simulink model "4sensors in a line"  (R2019a)
settings: Solver=FixedStepAuto  StartTime=0.0  StopTime=10.0  RelTol=1e-3
undefined symbols (not defined in the file or in its folder): Battery, GYRO, LME, LRLI, MODE, MSE, PING, RME, RRLI
libraries: legoev3lib x44, simulink x19, dspstat3 x5, fuzblock x3, dspmtrx3 x3, simulink_extras x1
(part 1 of 2)
settings Model: SimulationMode=external  ExtModeTrigDuration=2  Creator=dlharr12  LastModifiedBy=juana
settings SolverCC: PositivePriorityOrder=on
settings DataIOCC: ReturnWorkspaceOutputs=off
settings OptimizationCC: PassReuseOutputArgsAs=Individual arguments  MaxStackSize=64
settings DebuggingCC: ParameterTunabilityLossMsg=error  ArithmeticOperatorsInVariantConditions=warning
settings HardwareCC: ProdBitPerPointer=32  ProdBitPerSizeT=32  ProdBitPerPtrDiffT=32  ProdLargestAtomicInteger=Long  ProdWordSize=32  ProdHWDeviceType=ARM Compatible->ARM 9  UseEmbeddedCoderFeatures=off  UseSimulinkCoderFeatures=off
settings SFSimCC: SimUseLocalCustomCode=off  MATLABDynamicMemAlloc=off
settings RTWCC: SystemTargetFile=ert.tlc  HardwareBoard=LEGO MINDSTORMS EV3  TLCOptions="-aInlineSetEventsForThisBaseRateFcn=TLC_FALSE -aSuppressMultiTaskScheduler=TLC_FALSE  -aRateBasedStepFcn=0"  TemplateMakefile=ert_default_tmf  GenerateReport=on  RTWUseLocalCustomCode=off  Toolchain=Sourcery G++ Lite v2009q3  IncludeHyperlinkInReport=on  LaunchReport=on  GenerateTraceInfo=on  GenerateTraceReport=on  GenerateTraceReportSl=on  GenerateTraceReportSf=on  GenerateTraceReportEml=on
settings CodeAppCC: ForceParamTrailComments=on  IgnoreCustomStorageClasses=off  OperatorAnnotations=on  SimulinkDataObjDesc=on  SFDataObjDesc=on  InsertBlockDesc=on
settings ERTTargetCC: SupportContinuousTime=on  SupportNonInlinedSFcns=on  SupportVariableSizeSignals=on

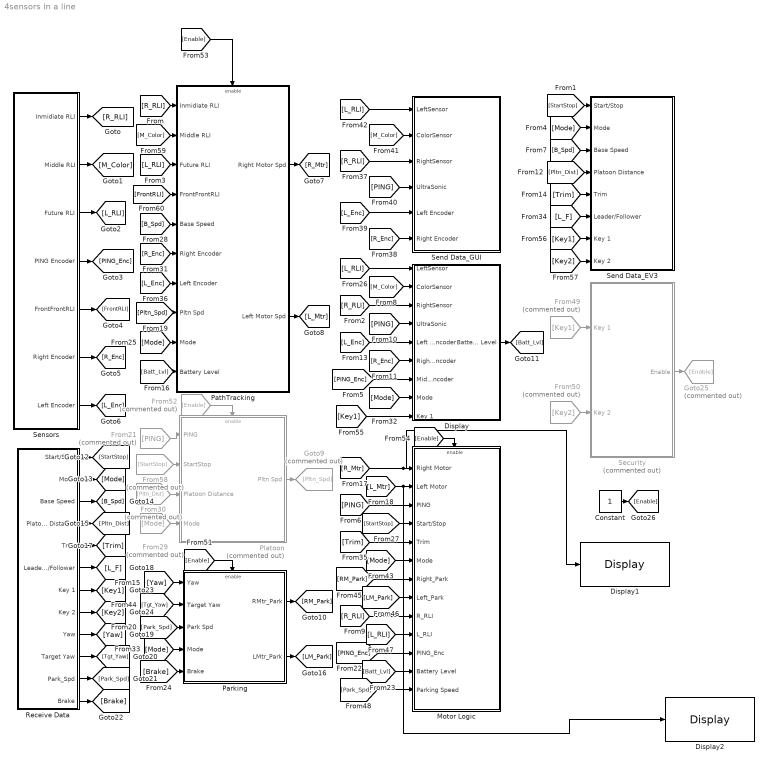
== system 4sensors in a line ==
  Constant : Constant
  Display : Subsystem
  Display1 : legoev3lib/Display  slcdStr=Rightm2  slcdLine=5  slcdFormat=Decimal
      settings: SourceProductName=Simulink Support Package for LEGO MINDSTORMS EV3 Hardware  SourceProductBaseCode=LEGOEV3
  Display2 : legoev3lib/Display  slcdStr=Leftm2  slcdLine=6  slcdFormat=Decimal
      settings: SourceProductName=Simulink Support Package for LEGO MINDSTORMS EV3 Hardware  SourceProductBaseCode=LEGOEV3
  From21 : From  Commented=on  GotoTag=PING
  From29 : From  Commented=on  GotoTag=Mode
  From30 : From  Commented=on  GotoTag=Pltn_Dist
  From49 : From  Commented=on  GotoTag=Key1
  From50 : From  Commented=on  GotoTag=Key2
  From52 : From  Commented=on  GotoTag=Enable
  From58 : From  Commented=on  GotoTag=StartStop
  Goto25 : Goto  Commented=on  GotoTag=Enable
  Goto9 : Goto  Commented=on  GotoTag=Pltn_Spd
  Motor Logic : Subsystem
  Parking : Subsystem
  PathTracking : Subsystem
  Platoon : Subsystem  Commented=on
  Receive Data : Subsystem
  Security : Subsystem  Commented=on
  Send Data_EV3 : Subsystem
  Send Data_GUI : Subsystem
  Sensors : Subsystem
  wires:
  Sensors/1(Inmidiate RLI) -> [R_RLI]
  Sensors/2(Middle RLI) -> [M_Color]
  Sensors/3(Future RLI) -> [L_RLI]
  Sensors/4(PING Encoder) -> [PING_Enc]
  Sensors/5(FrontFrontRLI) -> [FrontRLI]
  Sensors/6(Right Encoder) -> [R_Enc]
  Sensors/7(Left Encoder) -> [L_Enc]
  [R_Mtr] -> Display1/1, Motor Logic/1(Right Motor)
  [PING] -> Motor Logic/3(PING)
  [StartStop] -> Motor Logic/4(Start/Stop)
  Receive Data/2(Mode) -> [Mode]
  Receive Data/3(Base Speed) -> [B_Spd]
  Receive Data/4(Platoon Distance) -> [Pltn_Dist]
  [B_Spd] -> PathTracking/5(Base Speed)
  PathTracking/2(Left Motor Spd) -> [L_Mtr]
  From30/1 -> Platoon/3(Platoon Distance)
  Platoon/1(Pltn Spd) -> Goto9/1
  From29/1 -> Platoon/4(Mode)
  [L_RLI] -> PathTracking/3(Future RLI)
  [PING_Enc] -> Motor Logic/11(PING_Enc)
  From21/1 -> Platoon/1(PING)
  PathTracking/1(Right Motor Spd) -> [R_Mtr]
  [R_RLI] -> PathTracking/1(Inmidiate RLI)
  [R_Enc] -> Display/6(Right Encoder)
  [L_Enc] -> Display/5(Left Encoder)
  [PING] -> Display/4(UltraSonic)
  [L_RLI] -> Display/1(LeftSensor)
  [M_Color] -> Display/2(ColorSensor)
  [PING_Enc] -> Display/7(Middle Encoder)
  [R_RLI] -> Display/3(RightSensor)
  [Mode] -> Display/8(Mode)
  Receive Data/5(Trim) -> [Trim]
  [Trim] -> Motor Logic/5(Trim)
  [R_Enc] -> PathTracking/6(Right Encoder)
  [L_Enc] -> PathTracking/7(Left Encoder)
  [Pltn_Spd] -> PathTracking/8(Pltn Spd)
  [Mode] -> PathTracking/9(Mode)
  [R_Enc] -> Send Data_GUI/6(Right Encoder)
  [PING] -> Send Data_GUI/4(UltraSonic)
  [L_Enc] -> Send Data_GUI/5(Left Encoder)
  [R_RLI] -> Send Data_GUI/3(RightSensor)
  [M_Color] -> Send Data_GUI/2(ColorSensor)
  [L_RLI] -> Send Data_GUI/1(LeftSensor)
  [Mode] -> Motor Logic/6(Mode)
  Receive Data/6(Leader/Follower) -> [L_F]
  Parking/1(RMtr_Park) -> [RM_Park]
  Parking/2(LMtr_Park) -> [LM_Park]
  [RM_Park] -> Motor Logic/7(Right_Park)
  [LM_Park] -> Motor Logic/8(Left_Park)
  Receive Data/9(Yaw) -> [Yaw]
  Receive Data/10(Target Yaw) -> [Tgt_Yaw]
  [Yaw] -> Parking/1(Yaw)
  [Tgt_Yaw] -> Parking/2(Target Yaw)
  [Mode] -> Parking/4(Mode)
  [StartStop] -> Send Data_EV3/1(Start/Stop)
  [Mode] -> Send Data_EV3/2(Mode)
  [B_Spd] -> Send Data_EV3/3(Base Speed)
  [Pltn_Dist] -> Send Data_EV3/4(Platoon Distance)
  [Trim] -> Send Data_EV3/5(Trim)
  [L_F] -> Send Data_EV3/6(Leader/Follower)
  [R_RLI] -> Motor Logic/9(R_RLI)
  [L_RLI] -> Motor Logic/10(L_RLI)
  Display/1(Battery Level) -> [Batt_Lvl]
  [Batt_Lvl] -> PathTracking/10(Battery Level)
  Receive Data/11(Park_Spd) -> [Park_Spd]
  [Park_Spd] -> Parking/3(Park Spd)
  [Batt_Lvl] -> Motor Logic/12(Battery Level)
  Receive Data/12(Brake) -> [Brake]
  [Brake] -> Parking/5(Brake)
  [Park_Spd] -> Motor Logic/13(Parking Speed)
  Receive Data/7(Key 1) -> [Key1]
  Receive Data/8(Key 2) -> [Key2]
  From50/1 -> Security/2(Key 2)
  From49/1 -> Security/1(Key 1)
  Security/1(Enable) -> Goto25/1
  [Enable] -> Parking/Enable
  From52/1 -> Platoon/Enable
  [Enable] -> PathTracking/Enable
  [Enable] -> Motor Logic/Enable
  Receive Data/1(Start/Stop) -> [StartStop]
  [Key1] -> Display/9(Key 1)
  [Key1] -> Send Data_EV3/7(Key 1)
  [Key2] -> Send Data_EV3/8(Key 2)
  From58/1 -> Platoon/2(StartStop)
  Constant/1 -> [Enable]
  [M_Color] -> PathTracking/2(Middle RLI)
  [FrontRLI] -> PathTracking/4(FrontFrontRLI)
  [L_Mtr] -> Display2/1, Motor Logic/2(Left Motor)

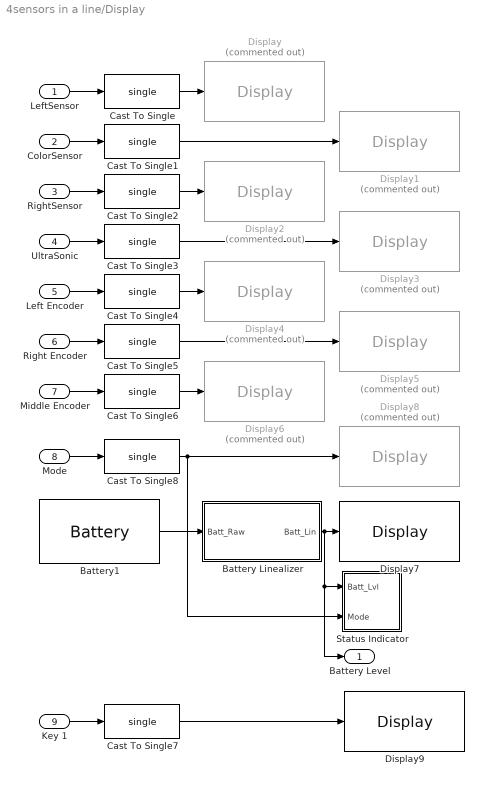
== system 4sensors in a line/Display ==
  LeftSensor : Inport
  ColorSensor : Inport  Port=2
  RightSensor : Inport  Port=3
  UltraSonic : Inport  Port=4
  Left Encoder : Inport  Port=5
  Right Encoder : Inport  Port=6
  Middle Encoder : Inport  Port=7
  Mode : Inport  Port=8
  Key 1 : Inport  Port=9
  Battery Linealizer : Subsystem
  Battery1 : legoev3lib/Battery  SampleTime=0.5
      settings: SourceProductName=Simulink Support Package for LEGO MINDSTORMS EV3 Hardware  SourceProductBaseCode=LEGOEV3
  Cast To Single{,1..8} (9 alike) : DataTypeConversion  OutDataTypeStr=single
  Display : legoev3lib/Display  Commented=on  slcdStr=LRLI:  slcdLine=1  slcdFormat=Decimal
      settings: SourceProductName=Simulink Support Package for LEGO MINDSTORMS EV3 Hardware  SourceProductBaseCode=LEGOEV3
  Display1 : legoev3lib/Display  Commented=on  slcdStr=GYRO:  slcdLine=2  slcdFormat=Decimal
      settings: SourceProductName=Simulink Support Package for LEGO MINDSTORMS EV3 Hardware  SourceProductBaseCode=LEGOEV3
  Display2 : legoev3lib/Display  Commented=on  slcdStr=RRLI:  slcdLine=3  slcdFormat=Decimal
      settings: SourceProductName=Simulink Support Package for LEGO MINDSTORMS EV3 Hardware  SourceProductBaseCode=LEGOEV3
  Display3 : legoev3lib/Display  Commented=on  slcdStr=PING:  slcdLine=4  slcdFormat=Decimal
      settings: SourceProductName=Simulink Support Package for LEGO MINDSTORMS EV3 Hardware  SourceProductBaseCode=LEGOEV3
  Display4 : legoev3lib/Display  Commented=on  slcdStr=LME:  slcdLine=5  slcdFormat=Decimal
      settings: SourceProductName=Simulink Support Package for LEGO MINDSTORMS EV3 Hardware  SourceProductBaseCode=LEGOEV3
  Display5 : legoev3lib/Display  Commented=on  slcdStr=RME:  slcdLine=6  slcdFormat=Decimal
      settings: SourceProductName=Simulink Support Package for LEGO MINDSTORMS EV3 Hardware  SourceProductBaseCode=LEGOEV3
  Display6 : legoev3lib/Display  Commented=on  slcdStr=MSE:  slcdLine=7  slcdFormat=Decimal
      settings: SourceProductName=Simulink Support Package for LEGO MINDSTORMS EV3 Hardware  SourceProductBaseCode=LEGOEV3
  Display7 : legoev3lib/Display  slcdStr=Battery:  slcdLine=9  slcdFormat=Decimal
      settings: SourceProductName=Simulink Support Package for LEGO MINDSTORMS EV3 Hardware  SourceProductBaseCode=LEGOEV3
  Display8 : legoev3lib/Display  Commented=on  slcdStr=MODE:  slcdLine=8  slcdFormat=Decimal
      settings: SourceProductName=Simulink Support Package for LEGO MINDSTORMS EV3 Hardware  SourceProductBaseCode=LEGOEV3
  Display9 : legoev3lib/Display  slcdStr=Key 1:  slcdLine=10  slcdFormat=Decimal
      settings: SourceProductName=Simulink Support Package for LEGO MINDSTORMS EV3 Hardware  SourceProductBaseCode=LEGOEV3
  Status Indicator : Subsystem
  Battery Level : Outport
  wires:
  ColorSensor/1 -> Cast To Single1/1
  LeftSensor/1 -> Cast To Single/1
  RightSensor/1 -> Cast To Single2/1
  UltraSonic/1 -> Cast To Single3/1
  Left Encoder/1 -> Cast To Single4/1
  Right Encoder/1 -> Cast To Single5/1
  Middle Encoder/1 -> Cast To Single6/1
  Cast To Single/1 -> Display/1
  Cast To Single1/1 -> Display1/1
  Cast To Single2/1 -> Display2/1
  Cast To Single3/1 -> Display3/1
  Cast To Single4/1 -> Display4/1
  Cast To Single5/1 -> Display5/1
  Cast To Single6/1 -> Display6/1
  Mode/1 -> Cast To Single8/1
  Cast To Single8/1 -> Status Indicator/2(Mode), Display8/1
  Battery1/1 -> Battery Linealizer/1(Batt_Raw)
  Battery Linealizer/1(Batt_Lin) -> Display7/1, Battery Level/1, Status Indicator/1(Batt_Lvl)
  Key 1/1 -> Cast To Single7/1
  Cast To Single7/1 -> Display9/1

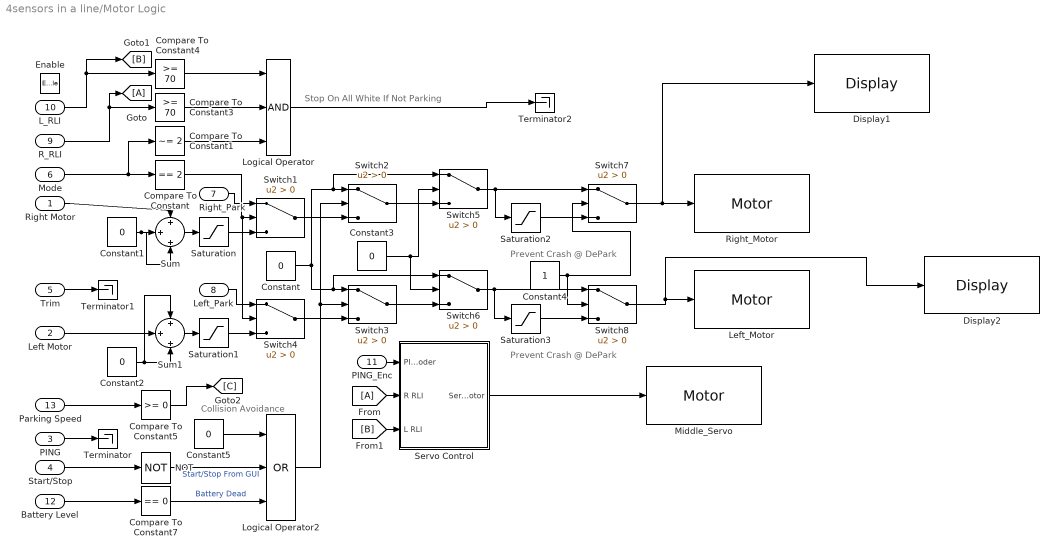
== system 4sensors in a line/Motor Logic ==
  note: Prevent Crash @ DePark
  note: Collision Avoidance
  note: Stop On All White If Not Parking
  note: Prevent Crash @ DePark
  Right Motor : Inport
  Left Motor : Inport  Port=2
  PING : Inport  Port=3
  Start/Stop : Inport  Port=4
  Trim : Inport  Port=5
  Mode : Inport  Port=6
  Right_Park : Inport  Port=7
  Left_Park : Inport  Port=8
  R_RLI : Inport  Port=9
  L_RLI : Inport  Port=10
  PING_Enc : Inport  Port=11
  Battery Level : Inport  Port=12
  Parking Speed : Inport  Port=13
  Enable : EnablePort
  Compare To Constant : simulink/Logic and Bit Operations/Compare To Constant  relop===  const=2  OutDataTypeStr=boolean
  Compare To Constant1 : simulink/Logic and Bit Operations/Compare To Constant  relop=~=  const=2  OutDataTypeStr=boolean
  Compare To Constant3 : simulink/Logic and Bit Operations/Compare To Constant  relop=>=  const=70  OutDataTypeStr=boolean
  Compare To Constant4 : simulink/Logic and Bit Operations/Compare To Constant  relop=>=  const=70  OutDataTypeStr=boolean
  Compare To Constant5 : simulink/Logic and Bit Operations/Compare To Constant  relop=>=  const=0  OutDataTypeStr=boolean
  Compare To Constant7 : simulink/Logic and Bit Operations/Compare To Constant  relop===  const=0  OutDataTypeStr=boolean
  Constant{,1..3,5} (5 alike) : Constant  Value=0
  Constant4 : Constant
  Display1 : legoev3lib/Display  slcdStr=Rightm3  slcdLine=7  slcdFormat=Decimal
      settings: SourceProductName=Simulink Support Package for LEGO MINDSTORMS EV3 Hardware  SourceProductBaseCode=LEGOEV3
  Display2 : legoev3lib/Display  slcdStr=Leftm3  slcdLine=8  slcdFormat=Decimal
      settings: SourceProductName=Simulink Support Package for LEGO MINDSTORMS EV3 Hardware  SourceProductBaseCode=LEGOEV3
  Left_Motor : legoev3lib/Motor  sportNumber=D  sstopAction=Brake
  Logical Operator : Logic  Inputs=3  AllPortsSameDT=off  OutDataTypeStr=boolean
  Logical Operator2 : Logic  Operator=OR  Inputs=3  AllPortsSameDT=off  OutDataTypeStr=boolean
  Middle_Servo : legoev3lib/Motor  sportNumber=C  sstopAction=Brake
  NOT : Logic  Operator=NOT  IconShape=distinctive  AllPortsSameDT=off  OutDataTypeStr=boolean
  Right_Motor : legoev3lib/Motor  sportNumber=A  sstopAction=Brake
  Saturation : Saturate  UpperLimit=100  LowerLimit=-100
  Saturation1 : Saturate  UpperLimit=100  LowerLimit=-100
  Saturation2 : Saturate  UpperLimit=0  LowerLimit=-100
  Saturation3 : Saturate  UpperLimit=0  LowerLimit=-100
  Servo Control : Subsystem
  Sum : Sum  Inputs=+|+|+
  Sum1 : Sum  Inputs=+|+|+
  Switch{1..8} (8 alike) : Switch  Criteria=u2 > Threshold
  Terminator : Terminator
  Terminator1 : Terminator
  Terminator2 : Terminator
  wires:
  Sum1/1 -> Saturation1/1
  Start/Stop/1 -> NOT/1
  NOT/1 -> Logical Operator2/2  "Start/Stop From GUI"
  Right Motor/1 -> Sum/1
  Sum/1 -> Saturation/1
  Left Motor/1 -> Sum1/2
  Mode/1 -> Compare To Constant1/1, Compare To Constant/1
  Saturation/1 -> Switch1/3
  Saturation1/1 -> Switch4/3
  Compare To Constant/1 -> Switch4/2, Switch1/2
  Right_Park/1 -> Switch1/1
  Left_Park/1 -> Switch4/1
  Logical Operator2/1 -> Switch3/2, Switch2/2
  Switch1/1 -> Switch2/3
  Switch4/1 -> Switch3/3
  Constant/1 -> Switch5/1, Switch2/1, Switch6/1, Switch3/1
  Constant1/1 -> Sum/3, Sum/2
  Constant2/1 -> Sum1/1, Sum1/3
  Switch2/1 -> Switch5/3
  Switch3/1 -> Switch6/3
  L_RLI/1 -> [B], Compare To Constant4/1
  R_RLI/1 -> [A], Compare To Constant3/1
  Servo Control/1(Servo Motor) -> Middle_Servo/1
  PING_Enc/1 -> Servo Control/1(PING Encoder)
  [A] -> Servo Control/2(R RLI)
  [B] -> Servo Control/3(L RLI)
  Compare To Constant1/1 -> Logical Operator/3
  Compare To Constant3/1 -> Logical Operator/2
  Compare To Constant4/1 -> Logical Operator/1
  Logical Operator/1 -> Terminator2/1
  Battery Level/1 -> Compare To Constant7/1
  Compare To Constant7/1 -> Logical Operator2/3  "Battery Dead"
  PING/1 -> Terminator/1
  Compare To Constant5/1 -> [C]
  Parking Speed/1 -> Compare To Constant5/1
  Saturation2/1 -> Switch7/3
  Switch8/1 -> Display2/1, Left_Motor/1
  Switch5/1 -> Saturation2/1, Switch7/1
  Saturation3/1 -> Switch8/3
  Constant4/1 -> Switch8/2, Switch7/2
  Switch6/1 -> Saturation3/1, Switch8/1
  Trim/1 -> Terminator1/1
  Constant3/1 -> Switch6/2, Switch5/2
  Constant5/1 -> Logical Operator2/1
  Switch7/1 -> Display1/1, Right_Motor/1

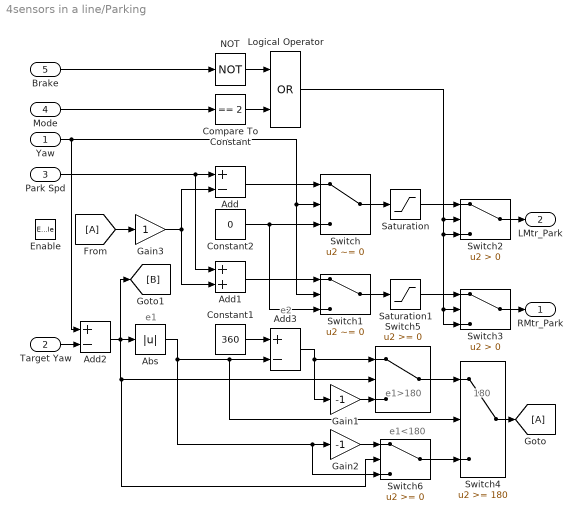
== system 4sensors in a line/Parking ==
  note: e1
  note: e2
  note: e1<180
  note: e1>180
  note: 180
  Yaw : Inport
  Target Yaw : Inport  Port=2
  Park Spd : Inport  Port=3
  Mode : Inport  Port=4
  Brake : Inport  Port=5
  Enable : EnablePort
  Abs : Abs
  Add : Sum  Inputs=+-
  Add1 : Sum
  Add2 : Sum  Inputs=+-
  Add3 : Sum  Inputs=+-
  Compare To Constant : simulink/Logic and Bit Operations/Compare To Constant  relop===  const=2  OutDataTypeStr=boolean
  Constant1 : Constant  Value=360
  Constant2 : Constant  Value=0
  Gain1 : Gain  Gain=-1
  Gain2 : Gain  Gain=-1
  Gain3 : Gain
  Logical Operator : Logic  Operator=OR  AllPortsSameDT=off  OutDataTypeStr=boolean
  NOT : Logic  Operator=NOT  IconShape=distinctive  AllPortsSameDT=off  OutDataTypeStr=boolean
  Saturation : Saturate  UpperLimit=60  LowerLimit=-60
  Saturation1 : Saturate  UpperLimit=60  LowerLimit=-60
  Switch : Switch  Criteria=u2 ~= 0
  Switch1 : Switch  Criteria=u2 ~= 0
  Switch2 : Switch  Criteria=u2 > Threshold
  Switch3 : Switch  Criteria=u2 > Threshold
  Switch4 : Switch  Threshold=180
  Switch5 : Switch
  Switch6 : Switch
  RMtr_Park : Outport
  LMtr_Park : Outport  Port=2
  wires:
  Mode/1 -> Compare To Constant/1
  Gain2/1 -> Switch6/1
  Target Yaw/1 -> Add2/2
  Add3/1 -> Gain1/1, Switch5/1
  Switch5/1 -> Switch4/1
  Switch6/1 -> Switch4/3
  Park Spd/1 -> Add1/1, Add/1
  Gain1/1 -> Switch5/3
  Gain3/1 -> Add/2, Add1/2
  Add2/1 -> [B], Switch6/2, Switch5/2, Abs/1
  Add/1 -> Switch/1
  Constant1/1 -> Add3/1
  Abs/1 -> Gain2/1, Switch6/3, Switch4/2, Add3/2
  Add1/1 -> Switch1/1
  Constant2/1 -> Switch1/3, Switch/3
  Yaw/1 -> Add2/1, Switch1/2, Switch/2
  Switch4/1 -> [A]
  [A] -> Gain3/1
  Switch2/1 -> LMtr_Park/1
  Switch3/1 -> RMtr_Park/1
  Compare To Constant/1 -> Logical Operator/2
  Logical Operator/1 -> Switch2/2, Switch2/3, Switch3/3, Switch3/2
  Brake/1 -> NOT/1
  NOT/1 -> Logical Operator/1
  Saturation/1 -> Switch2/1
  Saturation1/1 -> Switch3/1
  Switch/1 -> Saturation/1
  Switch1/1 -> Saturation1/1

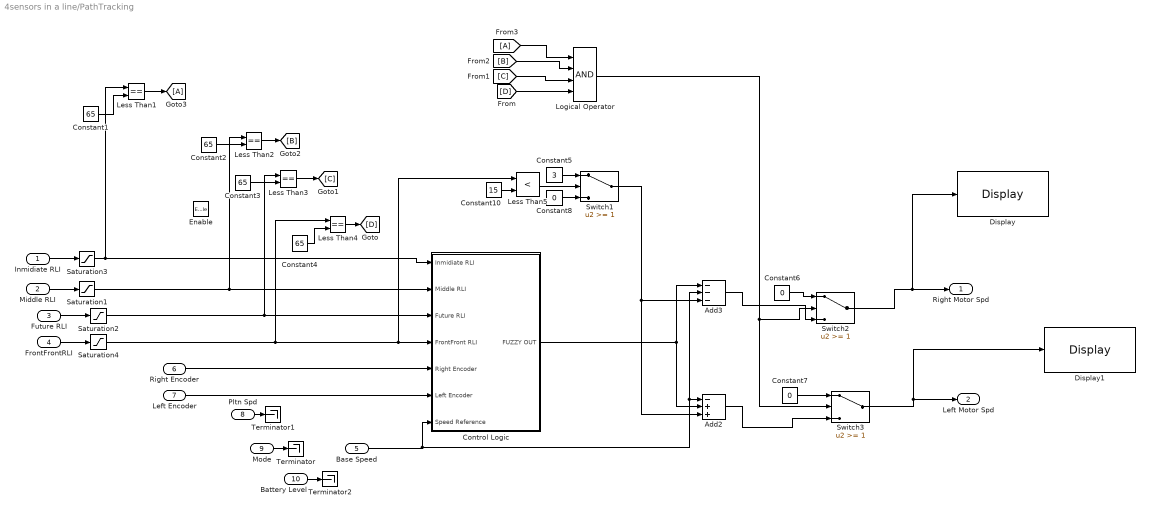
== system 4sensors in a line/PathTracking ==
  Inmidiate RLI : Inport
  Middle RLI : Inport  Port=2
  Future RLI : Inport  Port=3
  FrontFrontRLI : Inport  Port=4
  Base Speed : Inport  Port=5
  Right Encoder : Inport  Port=6
  Left Encoder : Inport  Port=7
  Pltn Spd : Inport  Port=8
  Mode : Inport  Port=9
  Battery Level : Inport  Port=10
  Enable : EnablePort
  Add2 : Sum  Inputs=-++
  Add3 : Sum  Inputs=---
  Constant{1..4} (4 alike) : Constant  Value=65
  Constant10 : Constant  Value=15
  Constant5 : Constant  Value=3
  Constant6 : Constant  Value=0
  Constant7 : Constant  Value=0
  Constant8 : Constant  Value=0
  Control Logic : Subsystem
  Display : legoev3lib/Display  slcdStr=Rightm  slcdLine=3  slcdFormat=Decimal
      settings: SourceProductName=Simulink Support Package for LEGO MINDSTORMS EV3 Hardware  SourceProductBaseCode=LEGOEV3
  Display1 : legoev3lib/Display  slcdStr=Leftm  slcdLine=4  slcdFormat=Decimal
      settings: SourceProductName=Simulink Support Package for LEGO MINDSTORMS EV3 Hardware  SourceProductBaseCode=LEGOEV3
  Less Than{1..4} (4 alike) : RelationalOperator  Operator===  OutDataTypeStr=boolean  RndMeth=Simplest
  Less Than5 : RelationalOperator  Operator=<  OutDataTypeStr=boolean  RndMeth=Simplest
  Logical Operator : Logic  Inputs=4  AllPortsSameDT=off  OutDataTypeStr=boolean
  Saturation{1..4} (4 alike) : Saturate  UpperLimit=65  LowerLimit=8
  Switch1 : Switch  Threshold=1
  Switch2 : Switch  Threshold=1
  Switch3 : Switch  Threshold=1
  Terminator : Terminator
  Terminator1 : Terminator
  Terminator2 : Terminator
  Right Motor Spd : Outport
  Left Motor Spd : Outport  Port=2
  wires:
  Future RLI/1 -> Saturation2/1
  Inmidiate RLI/1 -> Saturation3/1
  Control Logic/1(FUZZY OUT) -> Add2/2, Add3/1
  Right Encoder/1 -> Control Logic/5(Right Encoder)
  Left Encoder/1 -> Control Logic/6(Left Encoder)
  Mode/1 -> Terminator/1
  Base Speed/1 -> Control Logic/7(Speed Reference), Add3/2, Add2/1
  Battery Level/1 -> Terminator2/1
  Middle RLI/1 -> Saturation1/1
  Saturation4/1 -> Less Than5/1, Control Logic/4(FrontFront RLI), Less Than4/1
  Pltn Spd/1 -> Terminator1/1
  Constant10/1 -> Less Than5/2
  Constant5/1 -> Switch1/1
  Constant8/1 -> Switch1/3
  Less Than5/1 -> Switch1/2
  Switch1/1 -> Add3/3, Add2/3
  Saturation3/1 -> Control Logic/1(Inmidiate RLI), Less Than1/1
  Saturation1/1 -> Control Logic/2(Middle RLI), Less Than2/1
  Saturation2/1 -> Control Logic/3(Future RLI), Less Than3/1
  FrontFrontRLI/1 -> Saturation4/1
  Constant1/1 -> Less Than1/2
  Less Than1/1 -> [A]
  Constant2/1 -> Less Than2/2
  Less Than2/1 -> [B]
  Constant3/1 -> Less Than3/2
  Less Than3/1 -> [C]
  Constant4/1 -> Less Than4/2
  Less Than4/1 -> [D]
  Logical Operator/1 -> Switch3/2, Switch2/2
  Constant6/1 -> Switch2/1
  Constant7/1 -> Switch3/1
  Add2/1 -> Switch3/3
  Add3/1 -> Switch2/3
  Switch2/1 -> Display/1, Right Motor Spd/1
  Switch3/1 -> Display1/1, Left Motor Spd/1
  [D] -> Logical Operator/4
  [C] -> Logical Operator/3
  [B] -> Logical Operator/2
  [A] -> Logical Operator/1

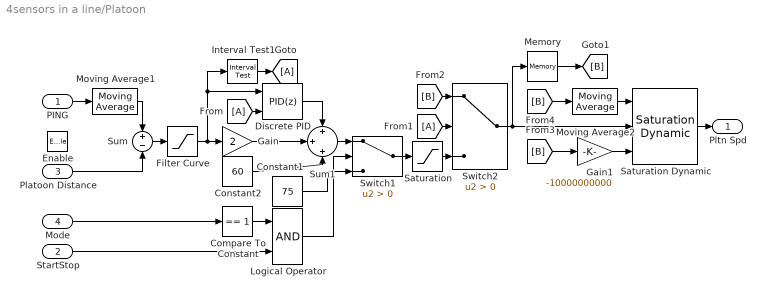
== system 4sensors in a line/Platoon ==
  PING : Inport
  StartStop : Inport  Port=2
  Platoon Distance : Inport  Port=3
  Mode : Inport  Port=4
  Enable : EnablePort
  Compare To Constant : simulink/Logic and Bit Operations/Compare To Constant  relop===  const=1  OutDataTypeStr=boolean
  Constant1 : Constant  Value=75
  Constant2 : Constant  Value=60
  Discrete PID : simulink/Continuous/PID Controller  Controller=PID  Form=Parallel  TimeDomain=Discrete-time  SampleTime=-1  IntegratorMethod=Forward Euler  FilterMethod=Forward Euler  ControllerParametersSource=internal  P=0  I=0.8  D=0  UseFilter=on  N=100  TunerSelectOption=Transfer Function Based (PID Tuner App)  InitialConditionSource=internal  InitialConditionForIntegrator=0  InitialConditionForFilter=0  DifferentiatorICPrevScaledInput=0  ExternalReset=level  TrackingMode=off  Kt=1  LimitOutput=off  UpperSaturationLimit=inf  LowerSaturationLimit=-inf  LinearizeAsGain=off  AntiWindupMode=none  Kb=1  POutMin=[]  POutMax=[]  IOutMin=[]  IOutMax=[]  DOutMin=[]  DOutMax=[]  NOutMin=[]  NOutMax=[]  SumOutMin=[]  SumOutMax=[]  SaturationOutMin=[]  SaturationOutMax=[]  PParamMin=[]  PParamMax=[]  IParamMin=[]  IParamMax=[]  DParamMin=[]  DParamMax=[]  NParamMin=[]  NParamMax=[]  KbParamMin=[]  KbParamMax=[]  KtParamMin=[]  KtParamMax=[]  KbOutMin=[]  KbOutMax=[]  KtOutMin=[]  KtOutMax=[]  IntegratorOutMin=[]  IntegratorOutMax=[]  FilterOutMin=[]  FilterOutMax=[]  SumI1OutMin=[]  SumI1OutMax=[]  SumI2OutMin=[]  SumI2OutMax=[]  SumI3OutMin=[]  SumI3OutMax=[]  SumI4OutMin=[]  SumI4OutMax=[]  SumDOutMin=[]  SumDOutMax=[]  DifferentiatorOutMin=[]  DifferentiatorOutMax=[]  FilterDiffOutCoefMin=[]  FilterDiffOutCoefMax=[]  ReciprocalOutMin=[]  ReciprocalOutMax=[]  SumDenOutMin=[]  SumDenOutMax=[]  SumNumOutMin=[]  SumNumOutMax=[]  DivideOutMin=[]  DivideOutMax=[]  IntegratorContinuousStateAttributes=''  IntegratorStateMustResolveToSignalObject=off  IntegratorRTWStateStorageClass=Auto  FilterContinuousStateAttributes=''  FilterStateMustResolveToSignalObject=off  FilterRTWStateStorageClass=Auto  ParallelPVariant=InternalParameters  IdealPVariant=Disabled  IVariant=InternalParameters  DVariant=InternalParameters  IntegratorVariant=Discrete  SatVariant=Disabled  AWVariant=Passthrough  PCopyVariant=Disabled  TRVariant=Disabled  FdbkBlocksVariant=Forward  IdealPFdbkVariant=Disabled  SatFdbkVariant=Disabled  DerivativeFilterVariant=ForwardEulerFilter  NVariant=InternalParameters  NCopyVariant=Disabled  FilterICVariant=InternalICsFilter  IntegratorICVariant=InternalICs  ExternalResetVariant=ExternalReset  TRSumVariant=Passthrough  SumFdbkVariant=Disabled  SumVariant=Sum_PID
  Filter Curve : Saturate  UpperLimit=30  LowerLimit=-30
  Gain : Gain  Gain=2
  Gain1 : Gain  Gain=-10000000000
  Interval Test1 : simulink/Logic and Bit Operations/Interval Test  IntervalClosedRight=on  uplimit=2  IntervalClosedLeft=on  lowlimit=-2  OutDataTypeStr=boolean
  Logical Operator : Logic  AllPortsSameDT=off  OutDataTypeStr=boolean
  Memory : Memory  InitialCondition=75
  Moving Average1 : dspstat3/Moving Average  Method=Sliding window  ForgettingFactorPort=off  SpecifyWindowLength=on  WindowLength=5  ForgettingFactor=0.9  SimulateUsing=Code generation
  Moving Average2 : dspstat3/Moving Average  Method=Sliding window  ForgettingFactorPort=off  SpecifyWindowLength=on  WindowLength=2000  ForgettingFactor=0.9  SimulateUsing=Code generation
  Saturation : Saturate  UpperLimit=100  LowerLimit=-100
  Saturation Dynamic : simulink/Discontinuities/Saturation Dynamic  OutMin=[]  OutMax=[]  OutDataTypeStr=Inherit: Same as second input  OutDataType=fixdt(1, 16)  OutScaling=2^-10  DoSatur=off
  Sum : Sum  Inputs=+|-
  Sum1 : Sum  Inputs=+|+|+
  Switch1 : Switch  Criteria=u2 > Threshold
  Switch2 : Switch  Criteria=u2 > Threshold
  Pltn Spd : Outport
  wires:
  PING/1 -> Moving Average1/1
  Platoon Distance/1 -> Sum/2
  Moving Average1/1 -> Sum/1
  Gain/1 -> Sum1/2
  Sum1/1 -> Switch1/1
  Saturation/1 -> Switch2/3
  Switch1/1 -> Saturation/1
  Mode/1 -> Compare To Constant/1
  Saturation Dynamic/1 -> Pltn Spd/1
  Interval Test1/1 -> [A]
  Filter Curve/1 -> Gain/1, Discrete PID/1, Interval Test1/1
  Discrete PID/1 -> Sum1/1
  Sum/1 -> Filter Curve/1
  Constant2/1 -> Sum1/3
  [A] -> Discrete PID/2
  [A] -> Switch2/2
  [B] -> Switch2/1
  Memory/1 -> [B]
  [B] -> Gain1/1
  [B] -> Moving Average2/1
  Switch2/1 -> Memory/1, Saturation Dynamic/2
  Moving Average2/1 -> Saturation Dynamic/1
  Gain1/1 -> Saturation Dynamic/3
  Logical Operator/1 -> Switch1/2
  Constant1/1 -> Switch1/3
  Compare To Constant/1 -> Logical Operator/1
  StartStop/1 -> Logical Operator/2

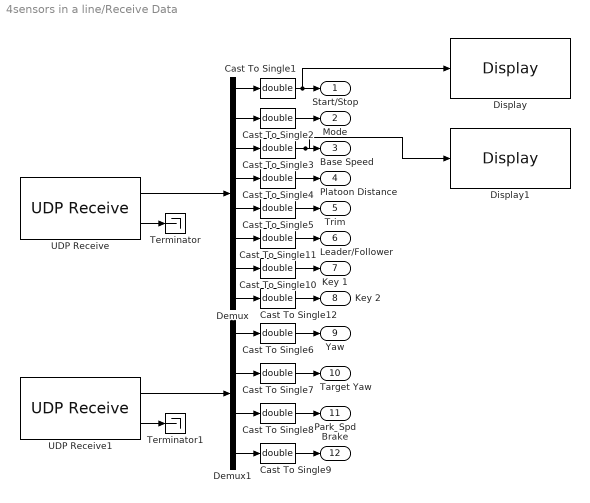
== system 4sensors in a line/Receive Data ==
  Cast To Single{1..12} (12 alike) : DataTypeConversion  OutDataTypeStr=double
  Demux : Demux  Outputs=8
  Demux1 : Demux
  Display : legoev3lib/Display  slcdStr=Start  slcdLine=1  slcdFormat=Decimal
      settings: SourceProductName=Simulink Support Package for LEGO MINDSTORMS EV3 Hardware  SourceProductBaseCode=LEGOEV3
  Display1 : legoev3lib/Display  slcdStr=BaseSpç  slcdLine=2  slcdFormat=Decimal
      settings: SourceProductName=Simulink Support Package for LEGO MINDSTORMS EV3 Hardware  SourceProductBaseCode=LEGOEV3
  Terminator : Terminator
  Terminator1 : Terminator
  UDP Receive : legoev3lib/UDP Receive  localURL='0.0.0.0'  localPort=PORT1  remoteURL='0.0.0.0'  remotePort=-1  recvBufferSize=8192  signalDatatype=int8  dims=8  isVarSize=off  showBlockingTime=off  blockingTime=0  sampletime=0.05  blockPlatform=LEGO EV3
      settings: SourceProductName=Simulink Support Package for LEGO MINDSTORMS EV3 Hardware  SourceProductBaseCode=LEGOEV3
  UDP Receive1 : legoev3lib/UDP Receive  localURL='0.0.0.0'  localPort=PORT2  remoteURL='0.0.0.0'  remotePort=-1  recvBufferSize=8192  signalDatatype=double  dims=4  isVarSize=off  showBlockingTime=off  blockingTime=0  sampletime=0.05  blockPlatform=LEGO EV3
      settings: SourceProductName=Simulink Support Package for LEGO MINDSTORMS EV3 Hardware  SourceProductBaseCode=LEGOEV3
  Start/Stop : Outport
  Mode : Outport  Port=2
  Base Speed : Outport  Port=3
  Platoon Distance : Outport  Port=4
  Trim : Outport  Port=5
  Leader/Follower : Outport  Port=6
  Key 1 : Outport  Port=7
  Key 2 : Outport  Port=8
  Yaw : Outport  Port=9
  Target Yaw : Outport  Port=10
  Park_Spd : Outport  Port=11
  Brake : Outport  Port=12
  wires:
  UDP Receive/2 -> Terminator/1
  UDP Receive/1 -> Demux/1
  Demux/1 -> Cast To Single1/1
  Demux/2 -> Cast To Single2/1
  Demux/3 -> Cast To Single3/1
  Demux/4 -> Cast To Single4/1
  Cast To Single2/1 -> Mode/1
  Cast To Single4/1 -> Platoon Distance/1
  Cast To Single3/1 -> Display1/1, Base Speed/1
  Cast To Single1/1 -> Display/1, Start/Stop/1
  Demux/5 -> Cast To Single5/1
  Cast To Single5/1 -> Trim/1
  UDP Receive1/2 -> Terminator1/1
  UDP Receive1/1 -> Demux1/1
  Demux1/1 -> Cast To Single6/1
  Cast To Single6/1 -> Yaw/1
  Cast To Single7/1 -> Target Yaw/1
  Demux1/2 -> Cast To Single7/1
  Demux/6 -> Cast To Single11/1
  Cast To Single11/1 -> Leader/Follower/1
  Demux1/3 -> Cast To Single8/1
  Cast To Single8/1 -> Park_Spd/1
  Demux1/4 -> Cast To Single9/1
  Cast To Single9/1 -> Brake/1
  Cast To Single10/1 -> Key 1/1
  Cast To Single12/1 -> Key 2/1
  Demux/8 -> Cast To Single12/1
  Demux/7 -> Cast To Single10/1

== system 4sensors in a line/Security ==
  Key 1 : Inport
  Key 2 : Inport  Port=2
  Button : legoev3lib/Button  buttonType=Down  sampleTime=0.1
      settings: SourceProductName=Simulink Support Package for LEGO MINDSTORMS EV3 Hardware  SourceProductBaseCode=LEGOEV3
  Cast To Boolean : DataTypeConversion  OutDataTypeStr=boolean
  Constant : Constant
  Constant1 : Constant  Value=0
  From Workspace : FromWorkspace  VariableName=key  OutDataTypeStr=double  SampleTime=0
  GreaterThanOrEqual : RelationalOperator  Operator===  OutDataTypeStr=boolean  RndMeth=Simplest
  GreaterThanOrEqual1 : RelationalOperator  Operator===  OutDataTypeStr=boolean  RndMeth=Simplest
  Logical Operator : Logic  AllPortsSameDT=off  OutDataTypeStr=boolean
  Logical Operator1 : Logic  AllPortsSameDT=off  OutDataTypeStr=boolean
  NOT : Logic  Operator=NOT  IconShape=distinctive  AllPortsSameDT=off  OutDataTypeStr=boolean
  NOT1 : Logic  Operator=NOT  IconShape=distinctive  AllPortsSameDT=off  OutDataTypeStr=boolean
  Security Alarm : Subsystem
  Submatrix : dspmtrx3/Submatrix  RowSpan=One row  RowStartMode=First  RowStartIndex=1  RowEndMode=Last  RowEndIndex=1  ColSpan=One column  ColStartMode=First  ColStartIndex=1  ColEndMode=Last  ColEndIndex=1
  Submatrix1 : dspmtrx3/Submatrix  RowSpan=One row  RowStartMode=Last  RowStartIndex=1  RowEndMode=Last  RowEndIndex=1  ColSpan=One column  ColStartMode=Last  ColStartIndex=1  ColEndMode=Last  ColEndIndex=1
  Switch : Switch  Criteria=u2 > Threshold
  Enable : Outport
  wires:
  Key 1/1 -> GreaterThanOrEqual/1
  Key 2/1 -> GreaterThanOrEqual1/1
  From Workspace/1 -> Submatrix1/1, Submatrix/1
  Submatrix/1 -> GreaterThanOrEqual/2
  Submatrix1/1 -> GreaterThanOrEqual1/2
  GreaterThanOrEqual/1 -> Logical Operator/1
  GreaterThanOrEqual1/1 -> Logical Operator/2
  Logical Operator/1 -> Switch/2
  Switch/1 -> Cast To Boolean/1, Enable/1
  Constant/1 -> Switch/1
  Constant1/1 -> Switch/3
  Cast To Boolean/1 -> NOT/1
  Button/1 -> NOT1/1
  NOT1/1 -> Logical Operator1/2
  NOT/1 -> Logical Operator1/1
  Logical Operator1/1 -> Security Alarm/Enable

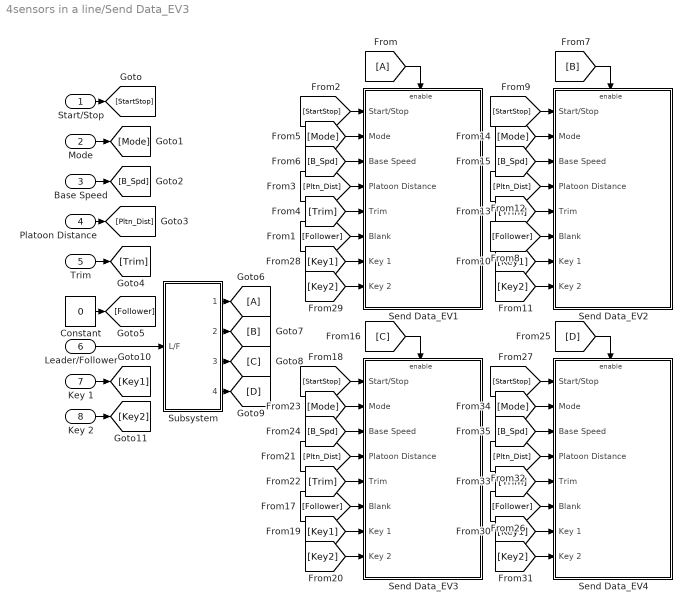
== system 4sensors in a line/Send Data_EV3 ==
  Start/Stop : Inport
  Mode : Inport  Port=2
  Base Speed : Inport  Port=3
  Platoon Distance : Inport  Port=4
  Trim : Inport  Port=5
  Leader/Follower : Inport  Port=6
  Key 1 : Inport  Port=7
  Key 2 : Inport  Port=8
  Constant : Constant  Value=0
  Send Data_EV1 : Subsystem
  Send Data_EV2 : Subsystem
  Send Data_EV3 : Subsystem
  Send Data_EV4 : Subsystem
  Subsystem : Subsystem
  wires:
  [Trim] -> Send Data_EV1/5(Trim)
  [Pltn_Dist] -> Send Data_EV1/4(Platoon Distance)
  [B_Spd] -> Send Data_EV1/3(Base Speed)
  [StartStop] -> Send Data_EV1/1(Start/Stop)
  [Mode] -> Send Data_EV1/2(Mode)
  Start/Stop/1 -> [StartStop]
  Mode/1 -> [Mode]
  Base Speed/1 -> [B_Spd]
  Platoon Distance/1 -> [Pltn_Dist]
  Trim/1 -> [Trim]
  Constant/1 -> [Follower]
  [Follower] -> Send Data_EV1/6(Blank)
  Leader/Follower/1 -> Subsystem/1(L/F)
  Subsystem/1(Active1) -> [A]
  Subsystem/2(Active2) -> [B]
  Subsystem/3(Active3) -> [C]
  Subsystem/4(Active4) -> [D]
  [A] -> Send Data_EV1/Enable
  Key 1/1 -> [Key1]
  Key 2/1 -> [Key2]
  [Key1] -> Send Data_EV1/7(Key 1)
  [Key2] -> Send Data_EV1/8(Key 2)
  [Key2] -> Send Data_EV2/8(Key 2)
  [Follower] -> Send Data_EV2/6(Blank)
  [B] -> Send Data_EV2/Enable
  [Trim] -> Send Data_EV2/5(Trim)
  [Pltn_Dist] -> Send Data_EV2/4(Platoon Distance)
  [StartStop] -> Send Data_EV2/1(Start/Stop)
  [B_Spd] -> Send Data_EV2/3(Base Speed)
  [Mode] -> Send Data_EV2/2(Mode)
  [Key1] -> Send Data_EV2/7(Key 1)
  [Key2] -> Send Data_EV3/8(Key 2)
  [Follower] -> Send Data_EV3/6(Blank)
  [C] -> Send Data_EV3/Enable
  [Trim] -> Send Data_EV3/5(Trim)
  [Pltn_Dist] -> Send Data_EV3/4(Platoon Distance)
  [StartStop] -> Send Data_EV3/1(Start/Stop)
  [B_Spd] -> Send Data_EV3/3(Base Speed)
  [Mode] -> Send Data_EV3/2(Mode)
  [Key1] -> Send Data_EV3/7(Key 1)
  [Key2] -> Send Data_EV4/8(Key 2)
  [Follower] -> Send Data_EV4/6(Blank)
  [D] -> Send Data_EV4/Enable
  [Trim] -> Send Data_EV4/5(Trim)
  [Pltn_Dist] -> Send Data_EV4/4(Platoon Distance)
  [StartStop] -> Send Data_EV4/1(Start/Stop)
  [B_Spd] -> Send Data_EV4/3(Base Speed)
  [Mode] -> Send Data_EV4/2(Mode)
  [Key1] -> Send Data_EV4/7(Key 1)

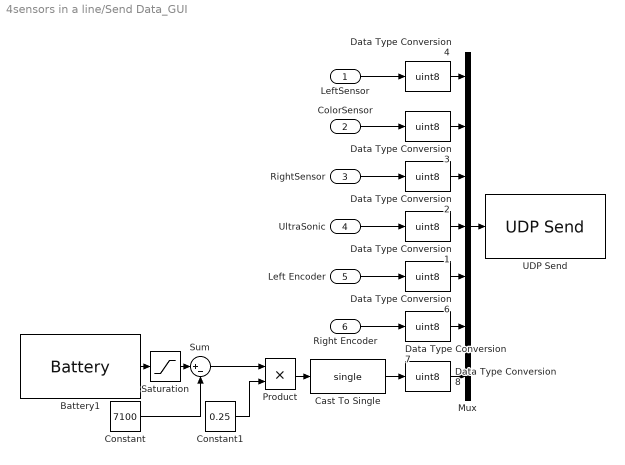
== system 4sensors in a line/Send Data_GUI ==
  LeftSensor : Inport
  ColorSensor : Inport  Port=2
  RightSensor : Inport  Port=3
  UltraSonic : Inport  Port=4
  Left Encoder : Inport  Port=5
  Right Encoder : Inport  Port=6
  Battery1 : legoev3lib/Battery  SampleTime=0.1
      settings: SourceProductName=Simulink Support Package for LEGO MINDSTORMS EV3 Hardware  SourceProductBaseCode=LEGOEV3
  Cast To Single : DataTypeConversion  OutDataTypeStr=single
  Constant : Constant  Value=7100
  Constant1 : Constant  Value=0.25
  Data Type Conversion{1..4,6..8} (7 alike) : DataTypeConversion  OutDataTypeStr=uint8
  Mux : Mux  Inputs=7
  Product : Product
  Saturation : Saturate  UpperLimit=7500  LowerLimit=7100
  Sum : Sum  Inputs=|+-
  UDP Send : legoev3lib/UDP Send  remoteURL=ip_address  remotePort=PORT1  localURL='0.0.0.0'  localPortSource=Automatically determine  localPort=PORT1  sampletime=-1  blockPlatform=LEGO EV3  separateLengthPort=0
      settings: SourceProductName=Simulink Support Package for LEGO MINDSTORMS EV3 Hardware  SourceProductBaseCode=LEGOEV3
  wires:
  UltraSonic/1 -> Data Type Conversion1/1
  RightSensor/1 -> Data Type Conversion2/1
  ColorSensor/1 -> Data Type Conversion3/1
  LeftSensor/1 -> Data Type Conversion4/1
  Mux/1 -> UDP Send/1
  Data Type Conversion1/1 -> Mux/4
  Data Type Conversion2/1 -> Mux/3
  Data Type Conversion3/1 -> Mux/2
  Data Type Conversion4/1 -> Mux/1
  Left Encoder/1 -> Data Type Conversion6/1
  Data Type Conversion6/1 -> Mux/5
  Right Encoder/1 -> Data Type Conversion7/1
  Data Type Conversion7/1 -> Mux/6
  Data Type Conversion8/1 -> Mux/7
  Cast To Single/1 -> Data Type Conversion8/1
  Constant/1 -> Sum/2
  Sum/1 -> Product/1
  Constant1/1 -> Product/2
  Product/1 -> Cast To Single/1
  Battery1/1 -> Saturation/1
  Saturation/1 -> Sum/1

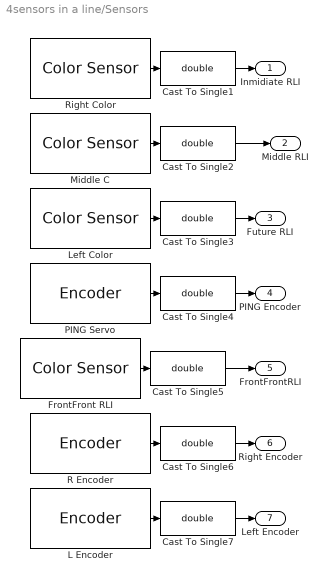
== system 4sensors in a line/Sensors ==
  Cast To Single{1..7} (7 alike) : DataTypeConversion  OutDataTypeStr=double
  "FrontFront RLI " : legoev3lib/Color Sensor  portNumber=4  mode=Reflected light intensity  sampleTime=0.01
      settings: SourceProductName=Simulink Support Package for LEGO MINDSTORMS EV3 Hardware  SourceProductBaseCode=LEGOEV3
  L Encoder : legoev3lib/Encoder  portNumber=D  opMode=No reset  sampleTime=0.01
      settings: SourceProductName=Simulink Support Package for LEGO MINDSTORMS EV3 Hardware  SourceProductBaseCode=LEGOEV3
  Left Color : legoev3lib/Color Sensor  portNumber=3  mode=Reflected light intensity  sampleTime=0.01
      settings: SourceProductName=Simulink Support Package for LEGO MINDSTORMS EV3 Hardware  SourceProductBaseCode=LEGOEV3
  Middle C : legoev3lib/Color Sensor  portNumber=2  mode=Reflected light intensity  sampleTime=0.01
      settings: SourceProductName=Simulink Support Package for LEGO MINDSTORMS EV3 Hardware  SourceProductBaseCode=LEGOEV3
  PING Servo : legoev3lib/Encoder  portNumber=C  opMode=No reset  sampleTime=0.01
      settings: SourceProductName=Simulink Support Package for LEGO MINDSTORMS EV3 Hardware  SourceProductBaseCode=LEGOEV3
  R Encoder : legoev3lib/Encoder  portNumber=A  opMode=No reset  sampleTime=0.01
      settings: SourceProductName=Simulink Support Package for LEGO MINDSTORMS EV3 Hardware  SourceProductBaseCode=LEGOEV3
  Right Color : legoev3lib/Color Sensor  portNumber=1  mode=Reflected light intensity  sampleTime=0.01
      settings: SourceProductName=Simulink Support Package for LEGO MINDSTORMS EV3 Hardware  SourceProductBaseCode=LEGOEV3
  Inmidiate RLI : Outport
  Middle RLI : Outport  Port=2
  Future RLI : Outport  Port=3
  PING Encoder : Outport  Port=4
  FrontFrontRLI : Outport  Port=5
  Right Encoder : Outport  Port=6
  Left Encoder : Outport  Port=7
  wires:
  R Encoder/1 -> Cast To Single6/1
  L Encoder/1 -> Cast To Single7/1
  PING Servo/1 -> Cast To Single4/1
  Middle C/1 -> Cast To Single2/1
  Right Color/1 -> Cast To Single1/1
  Left Color/1 -> Cast To Single3/1
  Cast To Single1/1 -> Inmidiate RLI/1
  Cast To Single6/1 -> Right Encoder/1
  Cast To Single3/1 -> Future RLI/1
  Cast To Single7/1 -> Left Encoder/1
  Cast To Single4/1 -> PING Encoder/1
  Cast To Single2/1 -> Middle RLI/1
  "FrontFront RLI "/1 -> Cast To Single5/1
  Cast To Single5/1 -> FrontFrontRLI/1

== system 4sensors in a line/Display/Battery Linealizer ==
  Batt_Raw : Inport
  Cast To Single9 : DataTypeConversion  OutDataTypeStr=single
  Constant : Constant  Value=7100
  Constant1 : Constant  Value=0.25
  Product : Product
  Saturation : Saturate  UpperLimit=7500  LowerLimit=7100
  Sum : Sum  Inputs=|+-
  Batt_Lin : Outport
  wires:
  Cast To Single9/1 -> Batt_Lin/1
  Saturation/1 -> Sum/1
  Sum/1 -> Product/1
  Constant/1 -> Sum/2
  Batt_Raw/1 -> Saturation/1
  Constant1/1 -> Product/2
  Product/1 -> Cast To Single9/1

== system 4sensors in a line/Display/Status Indicator ==
  Batt_Lvl : Inport
  Mode : Inport  Port=2
  Battery Alarm : legoev3lib/Speaker  sinputMode=Frequency and volume  sspeakerFreq=100  sspeakerVolume=50  sspeakerDuration=100
      settings: SourceProductName=Simulink Support Package for LEGO MINDSTORMS EV3 Hardware  SourceProductBaseCode=LEGOEV3
  Compare To Constant : simulink/Logic and Bit Operations/Compare To Constant  relop=<=  const=10  OutDataTypeStr=boolean
  Constant2 : Constant  Value=0
  Constant3 : Constant  Value=5000
  Constant4 : Constant  Value=100
  Status Light : Subsystem
  Switch : Switch  Criteria=u2 > Threshold
  wires:
  Constant3/1 -> Battery Alarm/1
  Constant4/1 -> Switch/1
  Constant2/1 -> Switch/3
  Batt_Lvl/1 -> Status Light/1(Battery), Compare To Constant/1
  Compare To Constant/1 -> Switch/2
  Switch/1 -> Battery Alarm/2
  Mode/1 -> Status Light/2(Mode)

== system 4sensors in a line/Motor Logic/Servo Control ==
  PING Encoder : Inport
  R RLI : Inport  Port=2
  L RLI : Inport  Port=3
  Abs3 : Abs
  Abs4 : Abs
  Constant3 : Constant  Value=0
  Constant4 : Constant
  Gain3 : Gain  Gain=1/3
  Gain4 : Gain  Gain=-1
  Interval Test1 : simulink/Logic and Bit Operations/Interval Test  IntervalClosedRight=on  uplimit=90  IntervalClosedLeft=on  lowlimit=15  OutDataTypeStr=boolean
  Moving Average1 : dspstat3/Moving Average  Method=Sliding window  ForgettingFactorPort=off  SpecifyWindowLength=on  WindowLength=15  ForgettingFactor=0.9  SimulateUsing=Code generation
  Sum2 : Sum  Inputs=+|-
  Switch5 : Switch  Criteria=u2 > Threshold  Threshold=5
  Switch6 : Switch  Criteria=u2 > Threshold  Threshold=40
  Switch7 : Switch  Criteria=u2 > Threshold
  Servo Motor : Outport
  wires:
  Gain3/1 -> Switch7/1
  PING Encoder/1 -> Abs4/1, Gain4/1
  Interval Test1/1 -> Switch7/2
  L RLI/1 -> Sum2/2
  Gain4/1 -> Switch5/1
  Switch5/1 -> [SL]
  Constant4/1 -> Switch6/1
  Constant3/1 -> Switch5/3
  R RLI/1 -> Sum2/1
  Abs3/1 -> Moving Average1/1
  Abs4/1 -> Switch5/2, Switch6/2
  [SL] -> Switch7/3
  Moving Average1/1 -> Interval Test1/1
  Switch6/1 -> Gain3/1
  Switch7/1 -> Servo Motor/1
  Sum2/1 -> Switch6/3, Abs3/1

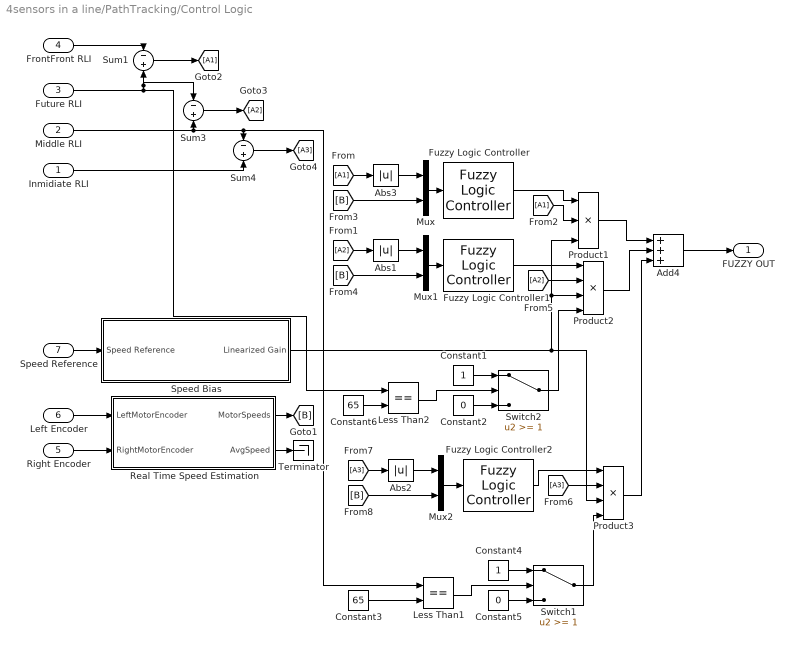
== system 4sensors in a line/PathTracking/Control Logic ==
  Inmidiate RLI : Inport
  Middle RLI : Inport  Port=2
  Future RLI : Inport  Port=3
  FrontFront RLI : Inport  Port=4
  Right Encoder : Inport  Port=5
  Left Encoder : Inport  Port=6
  Speed Reference : Inport  Port=7
  Abs1 : Abs
  Abs2 : Abs
  Abs3 : Abs
  Add4 : Sum  Inputs=+++
  Constant1 : Constant
  Constant2 : Constant  Value=0
  Constant3 : Constant  Value=65
  Constant4 : Constant
  Constant5 : Constant  Value=0
  Constant6 : Constant  Value=65
  Fuzzy Logic Controller : fuzblock/Fuzzy Logic  Controller  FIS='Fuzzy4P1.fis'  OutputSampleNumber=101  DataType=double  FuzzifiedInputs=off  RuleFiringStrengths=off  RuleOutputs=off  AggregatedOutputs=off  SimulateUsing=Interpreted execution  OutOfRangeInputValueMessage=warning  NoRuleFiredMessage=warning  EmptyOutputFuzzySetMessage=warning
  Fuzzy Logic Controller1 : fuzblock/Fuzzy Logic  Controller  FIS='Fuzzy4P2.fis'  OutputSampleNumber=101  DataType=double  FuzzifiedInputs=off  RuleFiringStrengths=off  RuleOutputs=off  AggregatedOutputs=off  SimulateUsing=Interpreted execution  OutOfRangeInputValueMessage=warning  NoRuleFiredMessage=warning  EmptyOutputFuzzySetMessage=warning
  Fuzzy Logic Controller2 : fuzblock/Fuzzy Logic  Controller  FIS='Fuzzy4P3.fis'  OutputSampleNumber=101  DataType=double  FuzzifiedInputs=off  RuleFiringStrengths=off  RuleOutputs=off  AggregatedOutputs=off  SimulateUsing=Interpreted execution  OutOfRangeInputValueMessage=warning  NoRuleFiredMessage=warning  EmptyOutputFuzzySetMessage=warning
  Less Than1 : RelationalOperator  Operator===  OutDataTypeStr=boolean  RndMeth=Simplest
  Less Than2 : RelationalOperator  Operator===  OutDataTypeStr=boolean  RndMeth=Simplest
  Mux : Mux  Inputs=2
  Mux1 : Mux  Inputs=2
  Mux2 : Mux  Inputs=2
  Product1 : Product  Inputs=3
  Product2 : Product  Inputs=4
  Product3 : Product  Inputs=4
  Real Time Speed Estimation : Subsystem
  Speed Bias : Subsystem
  Sum1 : Sum  Inputs=-|+
  Sum3 : Sum  Inputs=-|+
  Sum4 : Sum  Inputs=-|+
  Switch1 : Switch  Threshold=1
  Switch2 : Switch  Threshold=1
  Terminator : Terminator
  FUZZY OUT : Outport
  wires:
  Mux/1 -> Fuzzy Logic Controller/1
  Abs3/1 -> Mux/1
  Fuzzy Logic Controller/1 -> Product1/1
  Fuzzy Logic Controller1/1 -> Product2/1
  Mux1/1 -> Fuzzy Logic Controller1/1
  Abs1/1 -> Mux1/1
  Left Encoder/1 -> Real Time Speed Estimation/1(LeftMotorEncoder)
  Right Encoder/1 -> Real Time Speed Estimation/2(RightMotorEncoder)
  Speed Reference/1 -> Speed Bias/1(Speed Reference)
  Add4/1 -> FUZZY OUT/1
  Real Time Speed Estimation/2(AvgSpeed) -> Terminator/1
  [A1] -> Abs3/1
  [A2] -> Abs1/1
  [A1] -> Product1/2
  Real Time Speed Estimation/1(MotorSpeeds) -> [B]
  [B] -> Mux/2
  [B] -> Mux1/2
  Product2/1 -> Add4/2
  Product1/1 -> Add4/1
  Future RLI/1 -> Less Than2/1, Sum3/1, Sum1/2
  FrontFront RLI/1 -> Sum1/1
  Middle RLI/1 -> Less Than1/1, Sum4/1, Sum3/2
  Sum1/1 -> [A1]
  Sum3/1 -> [A2]
  Sum4/1 -> [A3]
  [A2] -> Product2/2
  Fuzzy Logic Controller2/1 -> Product3/1
  Product3/1 -> Add4/3
  Speed Bias/1(Linearized Gain) -> Product2/3, Product1/3, Product3/3
  [A3] -> Product3/2
  [B] -> Mux2/2
  [A3] -> Abs2/1
  Mux2/1 -> Fuzzy Logic Controller2/1
  Abs2/1 -> Mux2/1
  Constant5/1 -> Switch1/3
  Constant4/1 -> Switch1/1
  Less Than1/1 -> Switch1/2
  Switch1/1 -> Product3/4
  Constant3/1 -> Less Than1/2
  Inmidiate RLI/1 -> Sum4/2
  Constant1/1 -> Switch2/1
  Less Than2/1 -> Switch2/2
  Switch2/1 -> Product2/4
  Constant2/1 -> Switch2/3
  Constant6/1 -> Less Than2/2

== system 4sensors in a line/Security/Security Alarm ==
  Enable : EnablePort
  Battery Alarm : legoev3lib/Speaker  sinputMode=Frequency and volume  sspeakerFreq=100  sspeakerVolume=50  sspeakerDuration=100
      settings: SourceProductName=Simulink Support Package for LEGO MINDSTORMS EV3 Hardware  SourceProductBaseCode=LEGOEV3
  Constant2 : Constant  Value=100
  Constant3 : Constant  Value=0
  Constant4 : Constant  Value=2
  Gain : Gain  Gain=5000
  Gain1 : Gain  Gain=20
  Gain2 : Gain  Gain=-1
  Motor : legoev3lib/Motor  sportNumber=A  sstopAction=Brake
  Motor1 : legoev3lib/Motor  sportNumber=D  sstopAction=Brake
  Sine Wave1 : Sin  SineType=Sample based  Samples=100  SampleTime=0.01
  Status Light1 : legoev3lib/Status Light
      settings: SourceProductName=Simulink Support Package for LEGO MINDSTORMS EV3 Hardware  SourceProductBaseCode=LEGOEV3
  Switch1 : Switch  Criteria=u2 > Threshold
  Switch2 : Switch  Criteria=u2 > Threshold
  wires:
  Gain/1 -> Switch1/1, Switch1/2
  Sine Wave1/1 -> Switch2/2, Gain1/1, Gain/1
  Gain1/1 -> Motor1/1, Gain2/1
  Constant2/1 -> Battery Alarm/2
  Constant3/1 -> Switch2/3, Switch1/3
  Switch1/1 -> Battery Alarm/1
  Gain2/1 -> Motor/1
  Switch2/1 -> Status Light1/1
  Constant4/1 -> Switch2/1

== system 4sensors in a line/Send Data_EV3/Send Data_EV1 ==
  Start/Stop : Inport
  Mode : Inport  Port=2
  Base Speed : Inport  Port=3
  Platoon Distance : Inport  Port=4
  Trim : Inport  Port=5
  Blank : Inport  Port=6
  Key 1 : Inport  Port=7
  Key 2 : Inport  Port=8
  Enable : EnablePort
  Data Type Conversion{1..8} (8 alike) : DataTypeConversion  OutDataTypeStr=uint8
  Mux : Mux  Inputs=8
  UDP Send : legoev3lib/UDP Send  remoteURL='192.168.1.101'  remotePort=25001  localURL='0.0.0.0'  localPortSource=Automatically determine  localPort=Local_port  sampletime=-1  blockPlatform=LEGO EV3  separateLengthPort=0
      settings: SourceProductName=Simulink Support Package for LEGO MINDSTORMS EV3 Hardware  SourceProductBaseCode=LEGOEV3
  wires:
  Blank/1 -> Data Type Conversion6/1
  Data Type Conversion6/1 -> Mux/6
  Trim/1 -> Data Type Conversion5/1
  Data Type Conversion5/1 -> Mux/5
  Data Type Conversion1/1 -> Mux/4
  Base Speed/1 -> Data Type Conversion2/1
  Mux/1 -> UDP Send/1
  Data Type Conversion3/1 -> Mux/2
  Mode/1 -> Data Type Conversion3/1
  Data Type Conversion4/1 -> Mux/1
  Data Type Conversion2/1 -> Mux/3
  Start/Stop/1 -> Data Type Conversion4/1
  Platoon Distance/1 -> Data Type Conversion1/1
  Data Type Conversion8/1 -> Mux/8
  Data Type Conversion7/1 -> Mux/7
  Key 1/1 -> Data Type Conversion7/1
  Key 2/1 -> Data Type Conversion8/1

== system 4sensors in a line/Send Data_EV3/Send Data_EV2 ==
  Start/Stop : Inport
  Mode : Inport  Port=2
  Base Speed : Inport  Port=3
  Platoon Distance : Inport  Port=4
  Trim : Inport  Port=5
  Blank : Inport  Port=6
  Key 1 : Inport  Port=7
  Key 2 : Inport  Port=8
  Enable : EnablePort
  Data Type Conversion{1..8} (8 alike) : DataTypeConversion  OutDataTypeStr=uint8
  Mux : Mux  Inputs=8
  UDP Send : legoev3lib/UDP Send  remoteURL='192.168.1.102'  remotePort=25002  localURL='0.0.0.0'  localPortSource=Automatically determine  localPort=Local_port  sampletime=-1  blockPlatform=LEGO EV3  separateLengthPort=0
      settings: SourceProductName=Simulink Support Package for LEGO MINDSTORMS EV3 Hardware  SourceProductBaseCode=LEGOEV3
  wires:
  Blank/1 -> Data Type Conversion6/1
  Data Type Conversion6/1 -> Mux/6
  Trim/1 -> Data Type Conversion5/1
  Data Type Conversion5/1 -> Mux/5
  Data Type Conversion1/1 -> Mux/4
  Base Speed/1 -> Data Type Conversion2/1
  Mux/1 -> UDP Send/1
  Data Type Conversion3/1 -> Mux/2
  Mode/1 -> Data Type Conversion3/1
  Data Type Conversion4/1 -> Mux/1
  Data Type Conversion2/1 -> Mux/3
  Start/Stop/1 -> Data Type Conversion4/1
  Platoon Distance/1 -> Data Type Conversion1/1
  Data Type Conversion8/1 -> Mux/8
  Data Type Conversion7/1 -> Mux/7
  Key 1/1 -> Data Type Conversion7/1
  Key 2/1 -> Data Type Conversion8/1

== system 4sensors in a line/Send Data_EV3/Send Data_EV3 ==
  Start/Stop : Inport
  Mode : Inport  Port=2
  Base Speed : Inport  Port=3
  Platoon Distance : Inport  Port=4
  Trim : Inport  Port=5
  Blank : Inport  Port=6
  Key 1 : Inport  Port=7
  Key 2 : Inport  Port=8
  Enable : EnablePort
  Data Type Conversion{1..8} (8 alike) : DataTypeConversion  OutDataTypeStr=uint8
  Mux : Mux  Inputs=8
  UDP Send : legoev3lib/UDP Send  remoteURL='192.168.1.103'  remotePort=25003  localURL='0.0.0.0'  localPortSource=Automatically determine  localPort=Local_port  sampletime=-1  blockPlatform=LEGO EV3  separateLengthPort=0
      settings: SourceProductName=Simulink Support Package for LEGO MINDSTORMS EV3 Hardware  SourceProductBaseCode=LEGOEV3
  wires:
  Blank/1 -> Data Type Conversion6/1
  Data Type Conversion6/1 -> Mux/6
  Trim/1 -> Data Type Conversion5/1
  Data Type Conversion5/1 -> Mux/5
  Data Type Conversion1/1 -> Mux/4
  Base Speed/1 -> Data Type Conversion2/1
  Mux/1 -> UDP Send/1
  Data Type Conversion3/1 -> Mux/2
  Mode/1 -> Data Type Conversion3/1
  Data Type Conversion4/1 -> Mux/1
  Data Type Conversion2/1 -> Mux/3
  Start/Stop/1 -> Data Type Conversion4/1
  Platoon Distance/1 -> Data Type Conversion1/1
  Data Type Conversion8/1 -> Mux/8
  Data Type Conversion7/1 -> Mux/7
  Key 1/1 -> Data Type Conversion7/1
  Key 2/1 -> Data Type Conversion8/1

== system 4sensors in a line/Send Data_EV3/Send Data_EV4 ==
  Start/Stop : Inport
  Mode : Inport  Port=2
  Base Speed : Inport  Port=3
  Platoon Distance : Inport  Port=4
  Trim : Inport  Port=5
  Blank : Inport  Port=6
  Key 1 : Inport  Port=7
  Key 2 : Inport  Port=8
  Enable : EnablePort
  Data Type Conversion{1..8} (8 alike) : DataTypeConversion  OutDataTypeStr=uint8
  Mux : Mux  Inputs=8
  UDP Send : legoev3lib/UDP Send  remoteURL='192.168.1.104'  remotePort=25004  localURL='0.0.0.0'  localPortSource=Automatically determine  localPort=Local_port  sampletime=-1  blockPlatform=LEGO EV3  separateLengthPort=0
      settings: SourceProductName=Simulink Support Package for LEGO MINDSTORMS EV3 Hardware  SourceProductBaseCode=LEGOEV3
  wires:
  Blank/1 -> Data Type Conversion6/1
  Data Type Conversion6/1 -> Mux/6
  Trim/1 -> Data Type Conversion5/1
  Data Type Conversion5/1 -> Mux/5
  Data Type Conversion1/1 -> Mux/4
  Base Speed/1 -> Data Type Conversion2/1
  Mux/1 -> UDP Send/1
  Data Type Conversion3/1 -> Mux/2
  Mode/1 -> Data Type Conversion3/1
  Data Type Conversion4/1 -> Mux/1
  Data Type Conversion2/1 -> Mux/3
  Start/Stop/1 -> Data Type Conversion4/1
  Platoon Distance/1 -> Data Type Conversion1/1
  Data Type Conversion8/1 -> Mux/8
  Data Type Conversion7/1 -> Mux/7
  Key 1/1 -> Data Type Conversion7/1
  Key 2/1 -> Data Type Conversion8/1

== system 4sensors in a line/Send Data_EV3/Subsystem ==
  L/F : Inport
  Compare To Constant : simulink/Logic and Bit Operations/Compare To Constant  relop===  const=25001  OutDataTypeStr=boolean
  Compare To Constant1 : simulink/Logic and Bit Operations/Compare To Constant  relop===  const=25002  OutDataTypeStr=boolean
  Compare To Constant2 : simulink/Logic and Bit Operations/Compare To Constant  relop===  const=25003  OutDataTypeStr=boolean
  Compare To Constant3 : simulink/Logic and Bit Operations/Compare To Constant  relop===  const=25004  OutDataTypeStr=boolean
  Constant : Constant  Value=0
  From Workspace : FromWorkspace  VariableName=PORTM  OutDataTypeStr=double  SampleTime=0
  Submatrix : dspmtrx3/Submatrix  RowSpan=One row  RowStartMode=First  RowStartIndex=1  RowEndMode=Last  RowEndIndex=1  ColSpan=One column  ColStartMode=First  ColStartIndex=1  ColEndMode=Last  ColEndIndex=1
  Switch{,1..3} (4 alike) : Switch  Criteria=u2 > Threshold
  Active1 : Outport
  Active2 : Outport  Port=2
  Active3 : Outport  Port=3
  Active4 : Outport  Port=4
  wires:
  Switch/1 -> Active1/1
  Compare To Constant/1 -> Switch/2
  Switch1/1 -> Active2/1
  Switch2/1 -> Active3/1
  Switch3/1 -> Active4/1
  Compare To Constant1/1 -> Switch1/2
  Compare To Constant2/1 -> Switch2/2
  Compare To Constant3/1 -> Switch3/2
  L/F/1 -> Switch3/3, Switch2/3, Switch1/3, Switch/3
  Constant/1 -> Switch/1, Switch1/1, Switch2/1, Switch3/1
  From Workspace/1 -> Submatrix/1
  Submatrix/1 -> Compare To Constant3/1, Compare To Constant2/1, Compare To Constant1/1, Compare To Constant/1
